simulink model "subsistema_electromagnetico"  (R2020a)
settings: Solver=VariableStepAuto  StartTime=0.0  StopTime=10.0  RelTol=1e-3
model workspace: external: MATLAB File D:\Ferran\Facultad\UNCuyo\Meca\Automática y Máquinas Eléctricas\Proyecto final\matlab\parametros_y_especs\parametros_y_especif.m (data not in the file)
undefined symbols (not defined in the file): L_ls, lambda_m, Ld, Lq, Pp
settings Model: Creator=Ferran  LastModifiedBy=Ferran

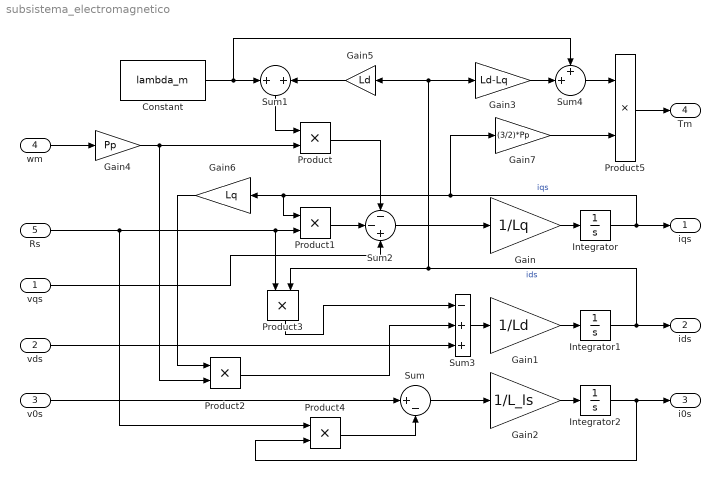
== system subsistema_electromagnetico ==
  vqs : Inport
  vds : Inport  Port=2
  v0s : Inport  Port=3
  wm : Inport  Port=4
  Rs : Inport  Port=5
  Constant : Constant  Value=lambda_m
  Gain : Gain  Gain=1/Lq
  Gain1 : Gain  Gain=1/Ld
  Gain2 : Gain  Gain=1/L_ls
  Gain3 : Gain  Gain=Ld-Lq
  Gain4 : Gain  Gain=Pp
  Gain5 : Gain  Gain=Ld
  Gain6 : Gain  Gain=Lq
  Gain7 : Gain  Gain=(3/2)*Pp
  Integrator : Integrator
  Integrator1 : Integrator
  Integrator2 : Integrator
  Product{,1..5} (6 alike) : Product
  Sum : Sum  Inputs=|+-
  Sum1 : Sum  Inputs=+|+
  Sum2 : Sum  Inputs=--+
  Sum3 : Sum  Inputs=-++
  Sum4 : Sum  Inputs=++|
  iqs : Outport
  ids : Outport  Port=2
  i0s : Outport  Port=3
  Tm : Outport  Port=4
  wires:
  Integrator/1 -> iqs/1, Gain7/1, Gain6/1, Product1/1  "iqs"
  Integrator2/1 -> Product4/2, i0s/1
  wm/1 -> Gain4/1
  Gain4/1 -> Product/2, Product2/2
  Integrator1/1 -> Product3/2, Gain5/1, Gain3/1, ids/1  "ids"
  Constant/1 -> Sum1/1, Sum4/1
  Gain5/1 -> Sum1/2
  Sum1/1 -> Product/1
  Rs/1 -> Product1/2, Product3/1, Product4/1
  Product/1 -> Sum2/1
  Product1/1 -> Sum2/2
  vqs/1 -> Sum2/3
  Sum2/1 -> Gain/1
  Gain/1 -> Integrator/1
  Gain1/1 -> Integrator1/1
  Gain2/1 -> Integrator2/1
  Gain6/1 -> Product2/1
  Product3/1 -> Sum3/1
  Product2/1 -> Sum3/2
  vds/1 -> Sum3/3
  Sum3/1 -> Gain1/1
  v0s/1 -> Sum/1
  Product4/1 -> Sum/2
  Sum/1 -> Gain2/1
  Gain3/1 -> Sum4/2
  Sum4/1 -> Product5/1
  Gain7/1 -> Product5/2
  Product5/1 -> Tm/1
